simulink model "DKSTDD_DK_TuanTuTietKiemNangLuong_SG_Y_Q_LQ"  (R2019a)
settings: Solver=VariableStepAuto  StartTime=0.0  StopTime=10.0  RelTol=1e-3
settings Model: Creator=Admin  LastModifiedBy=Admin

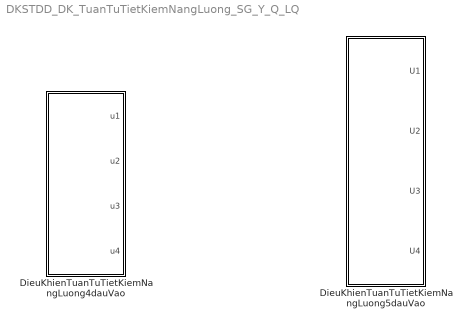
== system DKSTDD_DK_TuanTuTietKiemNangLuong_SG_Y_Q_LQ ==
  "DieuKhienTuanTuTietKiemNangLuong4dauVao " : Subsystem
  "DieuKhienTuanTuTietKiemNangLuong5dauVao " : Subsystem

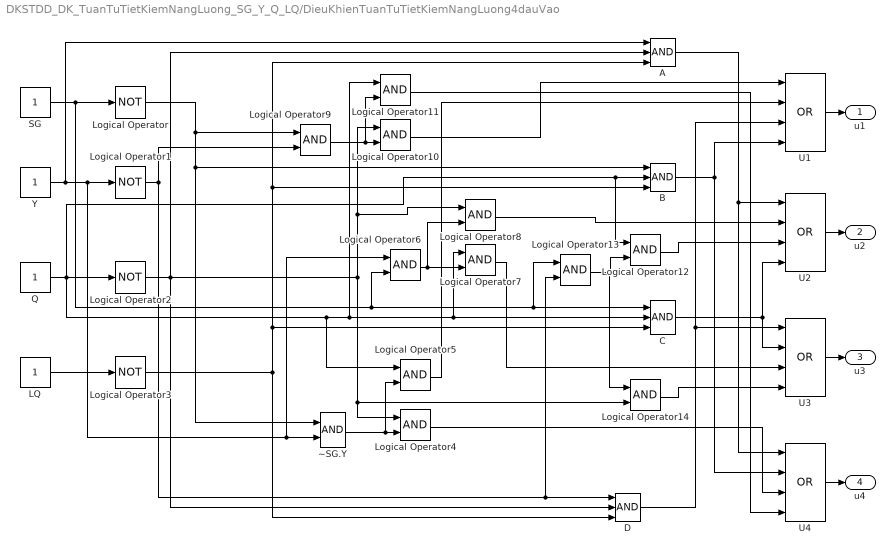
== system DKSTDD_DK_TuanTuTietKiemNangLuong_SG_Y_Q_LQ/DieuKhienTuanTuTietKiemNangLuong4dauVao  ==
  A : Logic  Inputs=3  AllPortsSameDT=off  OutDataTypeStr=boolean
  B : Logic  Inputs=3  AllPortsSameDT=off  OutDataTypeStr=boolean
  C : Logic  Inputs=3  AllPortsSameDT=off  OutDataTypeStr=boolean
  D : Logic  Inputs=3  AllPortsSameDT=off  OutDataTypeStr=boolean
  LQ : Constant
  Logical Operator{,1..3} (4 alike) : Logic  Operator=NOT  AllPortsSameDT=off  OutDataTypeStr=boolean
  Logical Operator{4..14} (11 alike) : Logic  AllPortsSameDT=off  OutDataTypeStr=boolean
  Q : Constant
  SG : Constant
  U{1..4} (4 alike) : Logic  Operator=OR  Inputs=4  AllPortsSameDT=off  OutDataTypeStr=boolean
  Y : Constant
  ~SG.Y : Logic  AllPortsSameDT=off  OutDataTypeStr=boolean
  u1 : Outport
  "u2 " : Outport  Port=2
  u3 : Outport  Port=3
  u4 : Outport  Port=4
  wires:
  Logical Operator3/1 -> D/3, C/3, B/3, A/3
  Logical Operator6/1 -> Logical Operator7/2, Logical Operator8/2
  Logical Operator9/1 -> Logical Operator11/2, Logical Operator10/2
  Q/1 -> C/2, Logical Operator7/1, Logical Operator11/1, Logical Operator5/1, Logical Operator12/1, B/2, Logical Operator2/1
  B/1 -> U4/2, U1/4
  Logical Operator8/1 -> U2/2
  Logical Operator10/1 -> U1/1
  Logical Operator/1 -> ~SG.Y/1, B/1, Logical Operator9/1
  A/1 -> U4/1, U2/1
  Logical Operator7/1 -> U3/3
  SG/1 -> C/1, Logical Operator13/1, Logical Operator6/2, Logical Operator/1
  Logical Operator2/1 -> Logical Operator4/1, Logical Operator14/2, Logical Operator10/1, Logical Operator8/1, D/2, A/2
  ~SG.Y/1 -> Logical Operator5/2, Logical Operator4/2
  LQ/1 -> Logical Operator3/1
  U4/1 -> u4/1
  Y/1 -> A/1, ~SG.Y/2, Logical Operator6/1, Logical Operator1/1
  Logical Operator5/1 -> U1/2
  D/1 -> U3/1, U1/3
  U3/1 -> u3/1
  Logical Operator1/1 -> Logical Operator9/2, Logical Operator13/2, D/1
  Logical Operator4/1 -> U4/3
  C/1 -> U3/2, U2/4
  Logical Operator14/1 -> U3/4
  Logical Operator11/1 -> U4/4
  Logical Operator13/1 -> Logical Operator14/1, Logical Operator12/2
  Logical Operator12/1 -> U2/3
  U2/1 -> "u2 "/1
  U1/1 -> u1/1

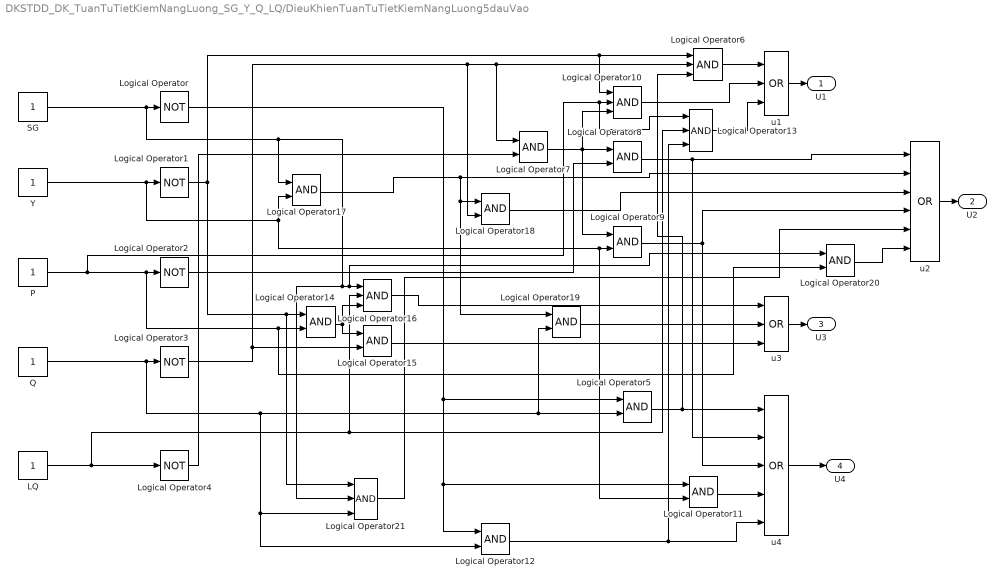
== system DKSTDD_DK_TuanTuTietKiemNangLuong_SG_Y_Q_LQ/DieuKhienTuanTuTietKiemNangLuong5dauVao  ==
  LQ : Constant
  Logical Operator{,1..4} (5 alike) : Logic  Operator=NOT  AllPortsSameDT=off  OutDataTypeStr=boolean
  Logical Operator{6,10,13,16,21} (5 alike) : Logic  Inputs=3  AllPortsSameDT=off  OutDataTypeStr=boolean
  Logical Operator{5,7..9,11..12,14..15,17..20} (12 alike) : Logic  AllPortsSameDT=off  OutDataTypeStr=boolean
  P : Constant
  Q : Constant
  SG : Constant
  Y : Constant
  u1 : Logic  Operator=OR  Inputs=3  AllPortsSameDT=off  OutDataTypeStr=boolean
  u2 : Logic  Operator=OR  Inputs=6  AllPortsSameDT=off  OutDataTypeStr=boolean
  u3 : Logic  Operator=OR  Inputs=3  AllPortsSameDT=off  OutDataTypeStr=boolean
  u4 : Logic  Operator=OR  Inputs=5  AllPortsSameDT=off  OutDataTypeStr=boolean
  U1 : Outport
  U2 : Outport  Port=2
  U3 : Outport  Port=3
  U4 : Outport  Port=4
  wires:
  SG/1 -> Logical Operator17/1, Logical Operator21/2, Logical Operator20/1, Logical Operator16/1, Logical Operator/1
  Logical Operator19/1 -> u3/2
  Logical Operator2/1 -> Logical Operator8/2
  Logical Operator/1 -> Logical Operator5/1, Logical Operator11/1, Logical Operator12/1
  Logical Operator11/1 -> u4/4
  Q/1 -> Logical Operator12/2, Logical Operator21/3, Logical Operator19/2, Logical Operator5/2, Logical Operator3/1
  P/1 -> Logical Operator13/1, Logical Operator10/2, Logical Operator20/2, Logical Operator14/2, Logical Operator2/1
  u4/1 -> U4/1
  Logical Operator20/1 -> u2/6
  Logical Operator18/1 -> u2/3
  Logical Operator17/1 -> Logical Operator18/1, Logical Operator19/1, u2/2
  Logical Operator5/1 -> u4/1, Logical Operator6/3
  Logical Operator3/1 -> Logical Operator18/2, Logical Operator6/2, Logical Operator7/1, Logical Operator15/2
  u1/1 -> U1/1
  Logical Operator21/1 -> u2/5
  Logical Operator9/1 -> u2/4, u4/3
  Logical Operator15/1 -> u3/3
  Logical Operator1/1 -> Logical Operator21/1, Logical Operator14/1, Logical Operator10/1, Logical Operator6/1
  Logical Operator8/1 -> u2/1, u4/2
  Logical Operator12/1 -> u4/5, Logical Operator13/3
  Logical Operator6/1 -> u1/1
  Logical Operator14/1 -> Logical Operator16/3, Logical Operator15/1
  LQ/1 -> Logical Operator16/2, Logical Operator13/2, Logical Operator4/1
  Logical Operator13/1 -> u1/3
  Y/1 -> Logical Operator17/2, Logical Operator11/2, Logical Operator9/2, Logical Operator1/1
  Logical Operator7/1 -> Logical Operator9/1, Logical Operator8/1, Logical Operator10/3
  Logical Operator16/1 -> u3/1
  Logical Operator4/1 -> Logical Operator7/2
  Logical Operator10/1 -> u1/2
  u3/1 -> U3/1
  u2/1 -> U2/1
